simulink model "filtering1"  (R2022b)
settings: Solver=FixedStepDiscrete  StartTime=0.0  StopTime=100  FixedStep=.1  RelTol=1e-3
values from neighbouring files (symbols this model uses):
  P0 = 1e2*eye(2)    [estimation2d.m]    (also in estimation3d.m = 1e2*eye(3); filtering1_s.m = V*diag([1 2])/V; filtering2_s.m = 1e1*eye(3); tst1.m = V*sqrt(D)*V.')
  R = (V /(sqrt(L))).'    [cellipse.m]    (also in estimation2d.m = V*D/V; estimation3d.m = V*D/V; filtering1_s.m = 3; filtering2_s.m = V*D/V)
  Ri = V*sqrt(L)    [cellipse.m]    (also in estimation2d.m = inv(R); estimation3d.m = inv(R); filtering1_s.m = inv(R); filtering2_s.m = inv(R))
  theta = 0:.05:2*pi    [cellipse.m]    (also in estimation2d.m = [8;-3]; estimation3d.m = [8;-3;4]; filtering1_s.m = [1.2, 3.4]; filtering2_s.m = [8;-3;15])
  xhat0 = [-5;-5]    [estimation2d.m]    (also in estimation3d.m = [-5;-5;0]; filtering1_s.m = [1;1]; filtering2_s.m = [0;0;0]; tst1.m)
libraries: dspinverses x2, ctrlSharedLib x1
settings Model: Creator=hp_desktop  LastModifiedBy=hp_desktop

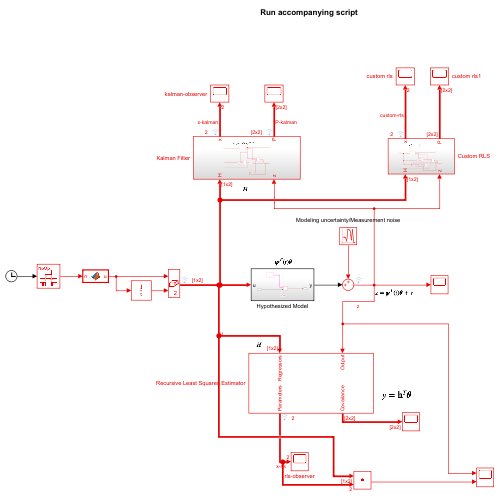
[thumbnail: Simulink's stored preview of the top-level diagram]
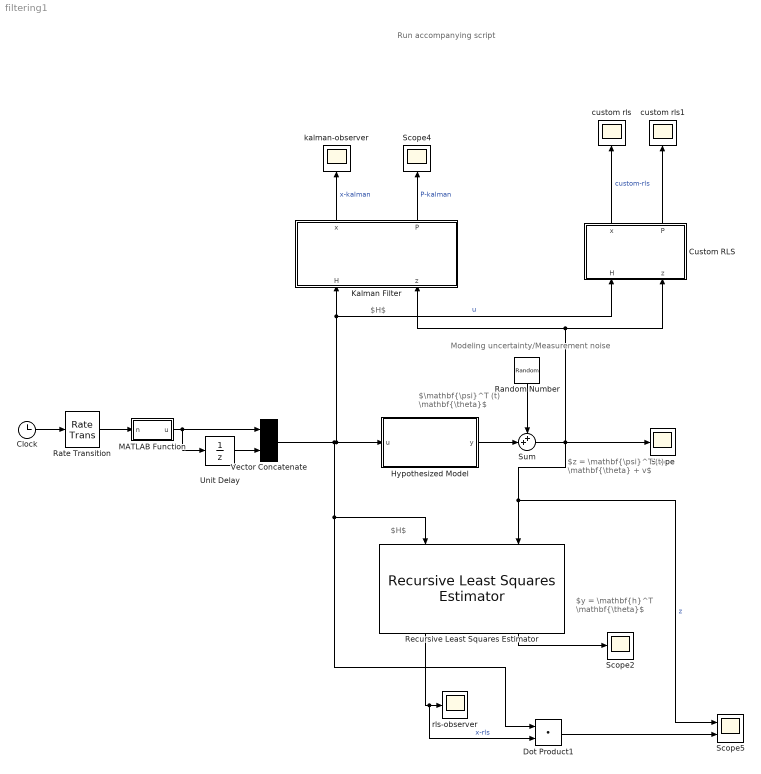
== system filtering1 ==
  note: Modeling uncertainty/Measurement noise
  note: Run accompanying script
  note: $H$
  note: $y = \mathbf{h}^T \mathbf{\theta}$
  note: $H$
  note: $z = \mathbf{\psi}^T (t) \mathbf{\theta} + v$
  note: $\mathbf{\psi}^T (t) \mathbf{\theta}$
  Clock : Clock
  Custom RLS : Subsystem
      settings: PortSchema="{\"entries\":[{\"content\":{\"sides\":[{\"content\":{\"connectorIds\":[]},\"type\":\"ConnectorPlacement.EquallySpacedRectSide\",\"uuid\":\"bee4a480-fac8-4835-b5c1-70eb87c43e95\"},{\"content\":{\"connectorIds\":[],\"side\":\"RIGHT\"},\"type\":\"ConnectorPlacement.EquallySpacedRectSide\",\"uuid\":\"cb84ae2e-f606-4d86-aba4-d3e87a068395\"},{\"content\":{\"connectorIds\":[\"Out1\",\"Out2\"],\"side\":\"TOP\"},\"type\":\"ConnectorPlacement.EquallySpacedRectSide\",\"uuid\":\"f12c143d-ef46-4cd1-bb91-64452094197f\"},{\"content\":{\"connectorIds\":[\"In1\",\"In2\"],\"side\":\"BOTTOM\"},\"type\":\"ConnectorPlacement.EquallySpacedRectSide\",\"uuid\":\"568da4d9-a657-45a3-b36e-930d4945feb0\"}]},\"type\":\"ConnectorPlacement.EquallySpacedConnector\",\"uuid\":\"8fe02375-4d00-45c9-82ce-5394bc2c2119\"}],\"packageUris\":[\"http://schema.mathworks.com/mf0/Connector/R2020b\"],\"version\":\"1.0\"}"
  Dot Product1 : DotProduct  OutDataTypeStr=Inherit: Inherit via internal rule
  Hypothesized Model : Subsystem
  Kalman Filter : Subsystem
  MATLAB Function : MATLAB Function  TreatAsAtomicUnit=on
  Random Number : RandomNumber  Variance=R  SampleTime=.1
  Rate Transition : RateTransition
  Recursive Least Squares Estimator : ctrlSharedLib/Recursive Least Squares Estimator  InitialEstimateSource=Internal  InitialParameterData=xhat0  P0=P0  InitialRegressors=0  InitialOutputs=0  History=Infinite  WindowLength=200  EstimationMethod=Forgetting Factor  AdaptationParameter=1  HasTimeVaryingAdaptationParameter=off  NormalizationBias=eps  OutputError=off  OutputP=on  AddEnablePort=off  InputProcessing=Sample-based  Ts=-1
      settings: LibrarySourceBlock=slident/Estimators/Recursive Least Squares Estimator
  Scope : Scope
  Scope2 : Scope
  Scope4 : Scope
  Scope5 : Scope  NumInputPorts=2
  Sum : Sum  Inputs=++|
  Unit Delay : UnitDelay  SampleTime=-1  HasFrameUpgradeWarning=on
  Vector Concatenate : Concatenate  Mode=Multidimensional array  ConcatenateDimension=2
  custom rls : Scope
  custom rls1 : Scope
  kalman-observer : Scope
  rls-observer : Scope
  wires:
  Clock/1 -> Rate Transition/1
  MATLAB Function/1(u) -> Unit Delay/1, Vector Concatenate/1
  Unit Delay/1 -> Vector Concatenate/2
  Vector Concatenate/1 -> Dot Product1/1, Recursive Least Squares Estimator/1, Hypothesized Model/1(u), Custom RLS/1(H), Kalman Filter/1(H)  "u"
  Sum/1 -> Custom RLS/2(z), Kalman Filter/2(z), Scope/1, Scope5/1, Recursive Least Squares Estimator/2  "z"
  Recursive Least Squares Estimator/1 -> Dot Product1/2, rls-observer/1  "x-rls"
  Rate Transition/1 -> MATLAB Function/1(n)
  Recursive Least Squares Estimator/2 -> Scope2/1
  Random Number/1 -> Sum/1
  Kalman Filter/1(x) -> kalman-observer/1  "x-kalman"
  Kalman Filter/2(P) -> Scope4/1  "P-kalman"
  Custom RLS/1(x) -> custom rls/1  "custom-rls"
  Custom RLS/2(P) -> custom rls1/1
  Dot Product1/1 -> Scope5/2
  Hypothesized Model/1(y) -> Sum/2

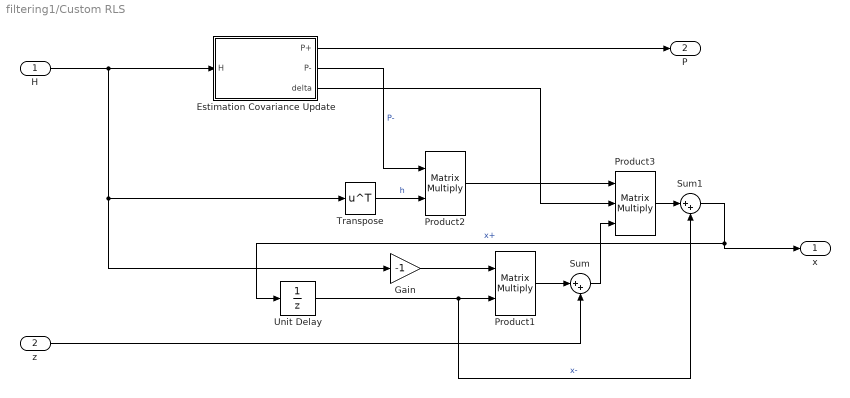
== system filtering1/Custom RLS ==
  H : Inport
  z : Inport  Port=2
  Estimation Covariance Update : Subsystem
  Gain : Gain  Gain=-1
  Product1 : Product  Multiplication=Matrix(*)
  Product2 : Product  Multiplication=Matrix(*)
  Product3 : Product  Inputs=3  Multiplication=Matrix(*)
  Sum : Sum  Inputs=|++
  Sum1 : Sum  Inputs=|++
  Transpose : Math  Operator=transpose
  Unit Delay : UnitDelay  SampleTime=-1  HasFrameUpgradeWarning=on
  x : Outport
  P : Outport  Port=2
  wires:
  Estimation Covariance Update/1(P+) -> P/1
  Unit Delay/1 -> Sum1/2, Product1/2  "x-"
  Sum1/1 -> x/1, Unit Delay/1  "x+"
  Transpose/1 -> Product2/2  "h"
  Product2/1 -> Product3/1
  Estimation Covariance Update/2(P-) -> Product2/1  "P-"
  H/1 -> Estimation Covariance Update/1(H), Gain/1, Transpose/1
  Gain/1 -> Product1/1
  Product1/1 -> Sum/1
  z/1 -> Sum/2
  Estimation Covariance Update/3(delta) -> Product3/2
  Sum/1 -> Product3/3
  Product3/1 -> Sum1/1

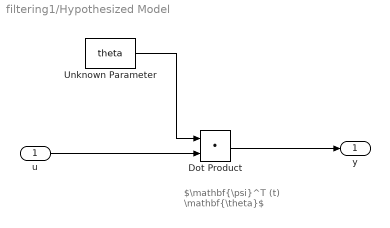
== system filtering1/Hypothesized Model ==
  note: $\mathbf{\psi}^T (t) \mathbf{\theta}$
  u : Inport
  Dot Product : DotProduct  OutDataTypeStr=Inherit: Inherit via internal rule
  Unknown Parameter : Constant  Value=theta  VectorParams1D=off
  y : Outport
  wires:
  Unknown Parameter/1 -> Dot Product/1
  u/1 -> Dot Product/2
  Dot Product/1 -> y/1

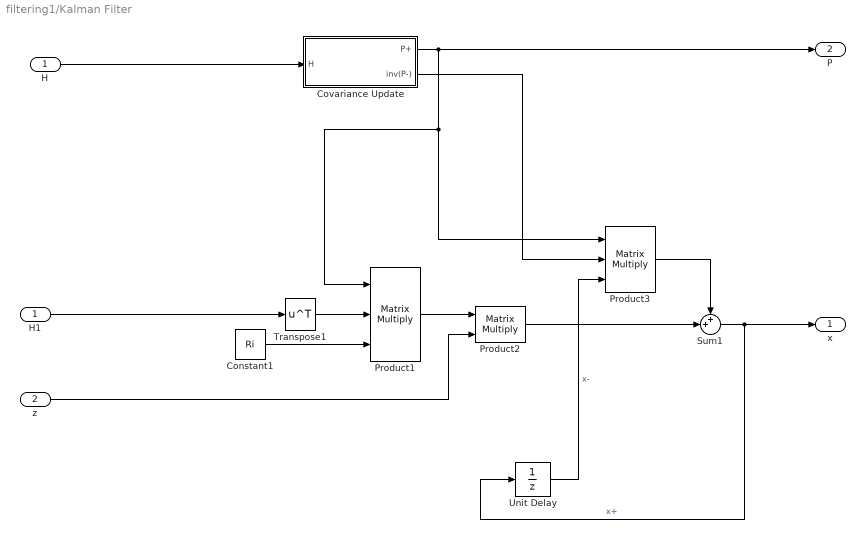
== system filtering1/Kalman Filter ==
  H : Inport
  z : Inport  Port=2
  Constant1 : Constant  Value=Ri  VectorParams1D=off
  Covariance Update : Subsystem
  H1 : InportShadow
  Product1 : Product  Inputs=3  Multiplication=Matrix(*)
  Product2 : Product  Multiplication=Matrix(*)
  Product3 : Product  Inputs=3  Multiplication=Matrix(*)
  Sum1 : Sum  Inputs=++|
  Transpose1 : Math  Operator=transpose
  Unit Delay : UnitDelay  InitialCondition=xhat0  SampleTime=-1  HasFrameUpgradeWarning=on
  x : Outport
  P : Outport  Port=2
  wires:
  Sum1/1 -> Unit Delay/1, x/1  "x+"
  Transpose1/1 -> Product1/2
  Constant1/1 -> Product1/3
  Product1/1 -> Product2/1
  z/1 -> Product2/2
  Unit Delay/1 -> Product3/3  "x-"
  Product3/1 -> Sum1/1
  Product2/1 -> Sum1/2
  H1/1 -> Transpose1/1
  Covariance Update/1(P+) -> P/1, Product1/1, Product3/1
  H/1 -> Covariance Update/1(H)
  Covariance Update/2(inv(P-)) -> Product3/2

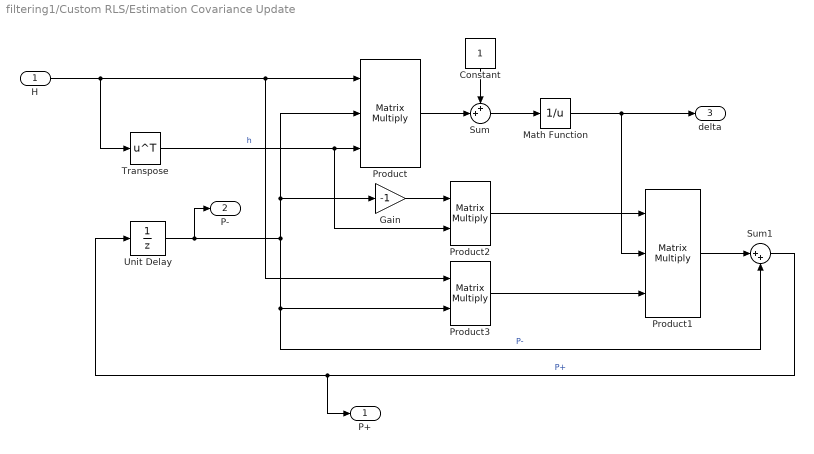
== system filtering1/Custom RLS/Estimation Covariance Update ==
  H : Inport
  Constant : Constant
  Gain : Gain  Gain=-1
  Math Function : Math  Operator=reciprocal
  Product : Product  Inputs=3  Multiplication=Matrix(*)
  Product1 : Product  Inputs=3  Multiplication=Matrix(*)
  Product2 : Product  Multiplication=Matrix(*)
  Product3 : Product  Multiplication=Matrix(*)
  Sum : Sum  Inputs=++|
  Sum1 : Sum  Inputs=|++
  Transpose : Math  Operator=transpose
  Unit Delay : UnitDelay  InitialCondition=diag([1 2])  SampleTime=-1  HasFrameUpgradeWarning=on
  P+ : Outport
  P- : Outport  Port=2
  delta : Outport  Port=3
  wires:
  Sum1/1 -> P+/1, Unit Delay/1  "P+"
  Unit Delay/1 -> P-/1, Sum1/2, Product3/2, Product/2, Gain/1  "P-"
  H/1 -> Transpose/1, Product3/1, Product/1
  Transpose/1 -> Product/3, Product2/2  "h"
  Product/1 -> Sum/2
  Constant/1 -> Sum/1
  Sum/1 -> Math Function/1
  Gain/1 -> Product2/1
  Product2/1 -> Product1/1
  Math Function/1 -> delta/1, Product1/2
  Product3/1 -> Product1/3
  Product1/1 -> Sum1/1

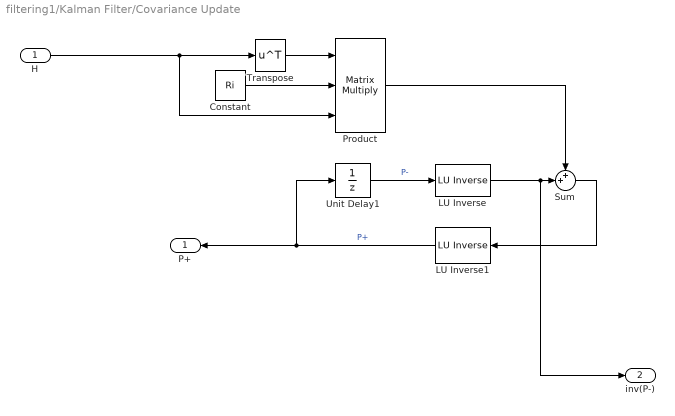
== system filtering1/Kalman Filter/Covariance Update ==
  H : Inport
  " LU Inverse" : dspinverses/ LU Inverse
  " LU Inverse1" : dspinverses/ LU Inverse
  Constant : Constant  Value=Ri  VectorParams1D=off
  Product : Product  Inputs=3  Multiplication=Matrix(*)
  Sum : Sum  Inputs=++|
  Transpose : Math  Operator=transpose
  Unit Delay1 : UnitDelay  InitialCondition=P0  SampleTime=-1  HasFrameUpgradeWarning=on
  P+ : Outport
  inv(P-) : Outport  Port=2
  wires:
  H/1 -> Product/3, Transpose/1
  Transpose/1 -> Product/1
  " LU Inverse"/1 -> inv(P-)/1, Sum/2
  " LU Inverse1"/1 -> Unit Delay1/1, P+/1  "P+"
  Constant/1 -> Product/2
  Product/1 -> Sum/1
  Unit Delay1/1 -> " LU Inverse"/1  "P-"
  Sum/1 -> " LU Inverse1"/1

== matlab function filtering1/MATLAB Function ==
  data: n input; u output
function u = fcn(n)

% u = sin(n) + cos(2*n) + exp(-.6*sin(3*n)) + cos(5*n) + sin(7*n) ...
%     + 1.2*sin(11*n) + cos(13*n) + cos(sin(.1*n)*n);
% ivec = [1 3 5 7 11 13 17 19 21];
% A = [0.2785    0.5469    0.9575    0.9649    0.1576    0.9706    0.9572    0.4854    0.8003];
ivec = [1 3 5 7 9 11];
A = [0.8147    0.9058    0.1270    0.9134    0.6324    0.0975];
u = 0;
j = 1;
for i =ivec
    u = u + A(j)*sin(.8*i*n);
    j = j +1;
end
u = u + exp(-.6*sin(3*n)) + cos(sin(.1*n)*n);
